simulink model "Engine"  (R2018a)
settings: Solver=VariableStepAuto  StartTime=0.0  StopTime=600  RelTol=1e-3
values from neighbouring files (symbols this model uses):
  fuel_density = 719.7    [IC_Engine.m]
  Initial_FL = 1    [IC_Engine.m]
  MFL = 5    [IC_Engine.m]
undefined symbols (not defined in the file or in its folder): fuelmap_fuel, fuelmap_spd, fuelmap_trq, map_spd, map_throttle, map_trq
libraries: simulink x2
settings Model: Creator=Saurabh Suman  LastModifiedBy=Saurabh Suman

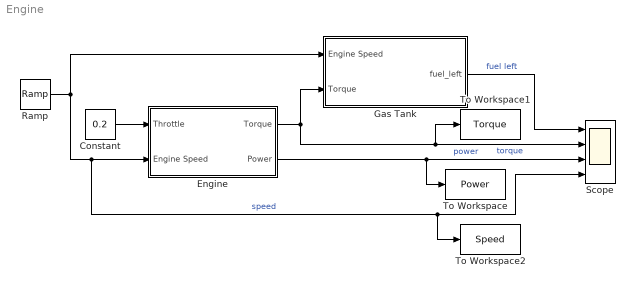
== system Engine ==
  Constant : Constant  Value=0.2
  Engine : Subsystem
  Gas Tank : Subsystem
  Ramp : simulink/Sources/Ramp  slope=1  start=0  InitialOutput=0
  Scope : Scope  NumInputPorts=4
  To Workspace : ToWorkspace  VariableName=Power  SaveFormat=Timeseries  SampleTime=-1
  To Workspace1 : ToWorkspace  VariableName=Torque  SaveFormat=Timeseries  SampleTime=-1
  To Workspace2 : ToWorkspace  VariableName=Speed  SaveFormat=Timeseries  SampleTime=-1
  wires:
  Engine/1(Torque) -> To Workspace1/1, Scope/2, Gas Tank/2(Torque)  "torque"
  Constant/1 -> Engine/1(Throttle)
  Ramp/1 -> To Workspace2/1, Scope/4, Engine/2(Engine Speed), Gas Tank/1(Engine Speed)  "speed"
  Engine/2(Power) -> To Workspace/1, Scope/3  "power"
  Gas Tank/1(fuel_left) -> Scope/1  "fuel left"

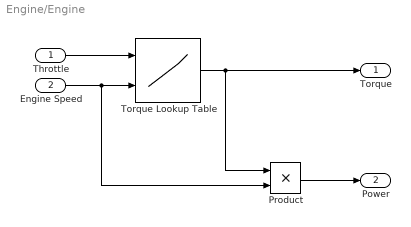
== system Engine/Engine ==
  Throttle : Inport
  Engine Speed : Inport  Port=2
  Product : Product
  Torque Lookup Table : Lookup_n-D  BreakpointsForDimension1=map_throttle  BreakpointsForDimension2=map_spd  Table=map_trq  InternalRulePriority=Speed  RndMeth=Simplest  InputSameDT=on
  Torque : Outport
  Power : Outport  Port=2
  wires:
  Throttle/1 -> Torque Lookup Table/1
  Torque Lookup Table/1 -> Torque/1, Product/1
  Engine Speed/1 -> Product/2, Torque Lookup Table/2
  Product/1 -> Power/1

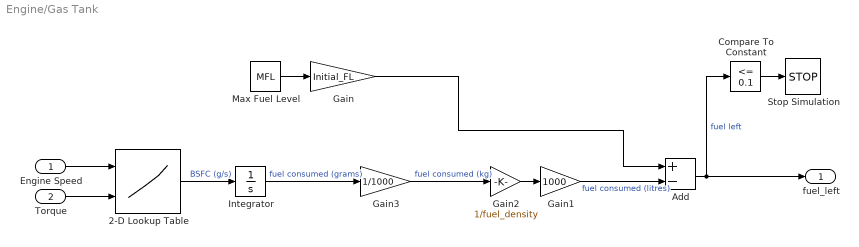
== system Engine/Gas Tank ==
  Engine Speed : Inport
  Torque : Inport  Port=2
  2-D Lookup Table : Lookup_n-D  BreakpointsForDimension1=fuelmap_spd  BreakpointsForDimension2=fuelmap_trq  Table=fuelmap_fuel  InternalRulePriority=Speed  RndMeth=Simplest  InputSameDT=on
  Add : Sum  Inputs=+-
  Compare To Constant : simulink/Logic and Bit Operations/Compare To Constant  relop=<=  const=0.1  OutDataTypeStr=boolean
  Gain : Gain  Gain=Initial_FL
  Gain1 : Gain  Gain=1000
  Gain2 : Gain  Gain=1/fuel_density
  Gain3 : Gain  Gain=1/1000
  Integrator : Integrator
  Max Fuel Level : Constant  Value=MFL
  Stop Simulation : Stop
  fuel_left : Outport
  wires:
  Integrator/1 -> Gain3/1  "fuel consumed (grams)"
  Gain3/1 -> Gain2/1  "fuel consumed (kg)"
  Gain2/1 -> Gain1/1
  Engine Speed/1 -> 2-D Lookup Table/1
  Gain/1 -> Add/1
  Gain1/1 -> Add/2  "fuel consumed (litres)"
  Torque/1 -> 2-D Lookup Table/2
  Add/1 -> fuel_left/1, Compare To Constant/1  "fuel left"
  Compare To Constant/1 -> Stop Simulation/1
  2-D Lookup Table/1 -> Integrator/1  "BSFC (g/s)"
  Max Fuel Level/1 -> Gain/1
